simulink model "sixDOF_hw6"  (R2015a)
settings: Solver=ode113  StartTime=0.0  StopTime=t_total  MaxStep=60  MinStep=0.1  RelTol=1e-3
values from neighbouring files (symbols this model uses):
  A0 = zeros(3,3)    [PS2.m]    (also in PS3.m = getDCM(triad1, triad2); PS4.m = getDCM(triad1, triad2); PS5.m = getDCM(triad1, triad2); PS7.m = getDCM(triad1, triad2))
  a0 = 6776    [PS1.m]    (also in PS4.m; PS5.m; PS7.m)
  A_b2p = S_top.DCM_B2P    [PS5.m]    (also in PS7.m)
  b_perturbs = 1    [PS5.m]    (also in PS7.m; PS8.m; PS9.m)
  bGravGrad = 1    [PS1.m]    (also in PS4.m; PS5.m; PS7.m; PS8.m)
  bNoise = 1    [PS6.m]    (also in PS7.m; PS8.m = 0; PS9.m = 0)
  e0 = 0.0004758    [PS1.m]    (also in PS4.m; PS5.m; PS7.m)
  I_principle = S_top.tauCM_P    [PS2.m]    (also in PS3.m; PS4.m; PS5.m; PS7.m)
  incl0 = 51.6397    [PS1.m]    (also in PS4.m = 0; PS5.m = 0; PS7.m = 0)
  J2 = 0    [PS1.m]    (also in PS4.m; PS5.m; PS7.m)
  M0 = [0 0 0]'    [PS2.m]    (also in PS3.m; PS4.m; PS5.m; PS7.m)
  mu = 3.986e14 / 1000^3    (= 398600)    [PS1.m]    (also in PS4.m; PS5.m; PS7.m)
  normalsList = [normalsList, chd.normals]    [S_top2Lists.m]
  nu0 = 0    [PS1.m]    (also in PS4.m; PS5.m; PS7.m)
  OMEGA0 = 106.0758    [PS1.m]    (also in PS4.m = 0; PS5.m = 0; PS7.m = 0)
  omega0 = 233.6745    [PS1.m]    (also in PS4.m = 0; PS5.m = 0; PS7.m = 0)
  Re = 6371    [PS1.m]    (also in PS4.m; PS5.m; PS7.m)
  surfaceAreasList = [surfaceAreasList; chd.surfaceAreas]    [S_top2Lists.m]
  surfaceCM_bodyList = [surfaceCM_bodyList, chd.surfaceCM_body]    [S_top2Lists.m]
  tOffset = 0    [PS5.m]    (also in PS7.m)
  UTC_0 = [06,02,2017]    [PS5.m]    (also in PS7.m)
  w0 = w0_28    [PS2.m]    (also in PS3.m = [0; 0; 10/180*pi*rand()]; PS4.m = w0 + 0.0007*[1 1 1]'; PS5.m = [0 -n0 0]'; PS7.m = [0 -2 0]')
  wEarth = [0 0 7.292116e-5]'    [PS5.m]    (also in PS7.m)
settings Model: Creator=Toby  LastModifiedBy=Toby
settings DataIOCC: SaveTime=off

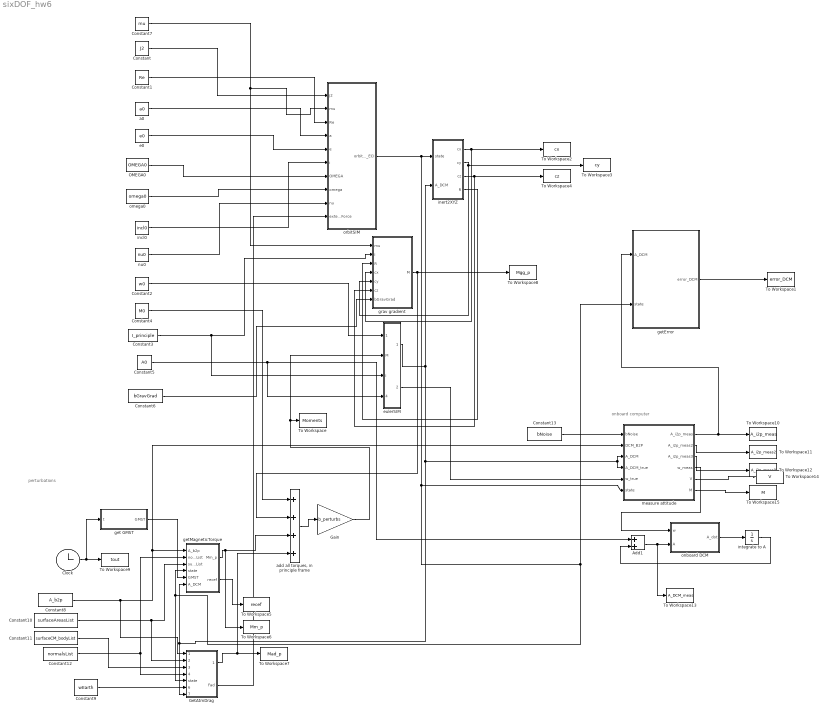
== system sixDOF_hw6 ==
  note: onboard computer
  note: perturbations
  Add1 : Sum
  Clock : Clock
  Constant : Constant  Value=J2
  Constant1 : Constant  Value=Re
  Constant10 : Constant  Value=surfaceAreasList
  Constant11 : Constant  Value=surfaceCM_bodyList
  Constant12 : Constant  Value=normalsList
  Constant13 : Constant  Value=bNoise
  Constant2 : Constant  Value=w0
  Constant3 : Constant  Value=I_principle
  Constant4 : Constant  Value=M0
  Constant5 : Constant  Value=A0
  Constant6 : Constant  Value=bGravGrad
  Constant7 : Constant  Value=mu
  Constant8 : Constant  Value=A_b2p
  Constant9 : Constant  Value=wEarth
  Gain : Gain  Gain=b_perturbs
  GetAtmDrag : MATLAB Function  TreatAsAtomicUnit=on
  OMEGA0 : Constant  Value=OMEGA0
  To Workspace : ToWorkspace  VariableName=Moments  SampleTime=-1
  To Workspace1 : ToWorkspace  VariableName=error_DCM  SampleTime=-1
  To Workspace10 : ToWorkspace  VariableName=A_i2p_meas  SampleTime=-1
  To Workspace11 : ToWorkspace  VariableName=A_i2p_meas2  SampleTime=-1
  To Workspace12 : ToWorkspace  VariableName=A_i2p_meas3  SampleTime=-1
  To Workspace13 : ToWorkspace  VariableName=A_DCM_meas  SampleTime=-1
  To Workspace14 : ToWorkspace  VariableName=V  SampleTime=-1
  To Workspace15 : ToWorkspace  VariableName=M  SampleTime=-1
  To Workspace2 : ToWorkspace  VariableName=cx  SampleTime=-1
  To Workspace3 : ToWorkspace  VariableName=cy  SampleTime=-1
  To Workspace4 : ToWorkspace  VariableName=cz  SampleTime=-1
  To Workspace5 : ToWorkspace  VariableName=recef  SampleTime=-1
  To Workspace6 : ToWorkspace  VariableName=Mm_p  SampleTime=-1
  To Workspace7 : ToWorkspace  VariableName=Mad_p  SampleTime=-1
  To Workspace8 : ToWorkspace  VariableName=Mgg_p  SampleTime=-1
  To Workspace9 : ToWorkspace  VariableName=tout  SampleTime=-1
  a0 : Constant  Value=a0
  "add all torques, in principle frame" : Sum  Inputs=++++
  e0 : Constant  Value=e0
  eulerSIM : Subsystem
  get GMST : Subsystem
  getError : MATLAB Function  TreatAsAtomicUnit=on
  getMagneticTorque : MATLAB Function  TreatAsAtomicUnit=on
  grav gradient : MATLAB Function  TreatAsAtomicUnit=on
  incl0 : Constant  Value=incl0
  inert2XYZ : MATLAB Function  TreatAsAtomicUnit=on
  integrate to A : Integrator
  measure attitude : MATLAB Function  TreatAsAtomicUnit=on
  nu0 : Constant  Value=nu0
  omega0 : Constant  Value=omega0
  onboard DCM : MATLAB Function  TreatAsAtomicUnit=on
  orbitSIM : Subsystem
  wires:
  Constant7/1 -> grav gradient/1(mu), orbitSIM/2(mu)
  Constant/1 -> orbitSIM/1(j2)
  Constant1/1 -> orbitSIM/3(Re)
  a0/1 -> orbitSIM/4(a)
  e0/1 -> orbitSIM/5(e)
  OMEGA0/1 -> orbitSIM/7(OMEGA)
  omega0/1 -> orbitSIM/8(omega)
  incl0/1 -> orbitSIM/6(i)
  nu0/1 -> orbitSIM/9(nu)
  Constant2/1 -> eulerSIM/1(w0)
  Constant3/1 -> grav gradient/2(I), eulerSIM/3(I)
  Constant5/1 -> Add1/1, eulerSIM/4(A0)
  inert2XYZ/1(cx) -> grav gradient/4(cx), To Workspace2/1
  inert2XYZ/2(cy) -> To Workspace3/1, grav gradient/5(cy)
  inert2XYZ/4(R) -> grav gradient/3(R)
  inert2XYZ/3(cz) -> To Workspace4/1, grav gradient/6(cz)
  Constant6/1 -> grav gradient/7(bGravGrad)
  Gain/1 -> eulerSIM/2(M), To Workspace/1
  GetAtmDrag/2(Fad) -> orbitSIM/10(externalForce)
  getError/1(error_DCM) -> To Workspace1/1
  grav gradient/1(M) -> "add all torques, in principle frame"/2, To Workspace8/1
  orbitSIM/1(orbit_state_ECI) -> measure attitude/6(state), getMagneticTorque/4(state), GetAtmDrag/5(state), getError/2(state), inert2XYZ/1(state)
  eulerSIM/1(A_DCM) -> inert2XYZ/2(A_DCM), measure attitude/4(A_DCM_true), measure attitude/3(A_DCM), getMagneticTorque/6(A_DCM), GetAtmDrag/7(A_DCM)
  "add all torques, in principle frame"/1 -> Gain/1
  Clock/1 -> get GMST/1(t), To Workspace9/1
  Constant8/1 -> measure attitude/2(DCM_B2P), getMagneticTorque/1(A_b2p), GetAtmDrag/1(A_b2p)
  GetAtmDrag/1(Mad_p) -> To Workspace7/1, "add all torques, in principle frame"/4
  Constant9/1 -> GetAtmDrag/6(wEarth)
  get GMST/1(GMST) -> getMagneticTorque/5(GMST)
  getMagneticTorque/2(recef) -> To Workspace5/1
  getMagneticTorque/1(Mm_p) -> "add all torques, in principle frame"/3, To Workspace6/1
  Constant12/1 -> getMagneticTorque/2(normalsList), GetAtmDrag/4(normalsList)
  Constant11/1 -> GetAtmDrag/3(surfaceCM_bodyList)
  Constant10/1 -> getMagneticTorque/3(surfaceAreasList), GetAtmDrag/2(surfaceAreasList)
  Constant4/1 -> "add all torques, in principle frame"/1
  onboard DCM/1(A_dot) -> integrate to A/1
  integrate to A/1 -> Add1/2
  Add1/1 -> To Workspace13/1, onboard DCM/2(A)
  measure attitude/4(w_meas) -> onboard DCM/1(w)
  measure attitude/1(A_i2p_meas) -> getError/1(A_DCM), To Workspace10/1
  measure attitude/2(A_i2p_meas2) -> To Workspace11/1
  measure attitude/3(A_i2p_meas3) -> To Workspace12/1
  Constant13/1 -> measure attitude/1(bNoise)
  eulerSIM/2(w_true) -> measure attitude/5(w_true)
  measure attitude/6(M) -> To Workspace15/1
  measure attitude/5(V) -> To Workspace14/1

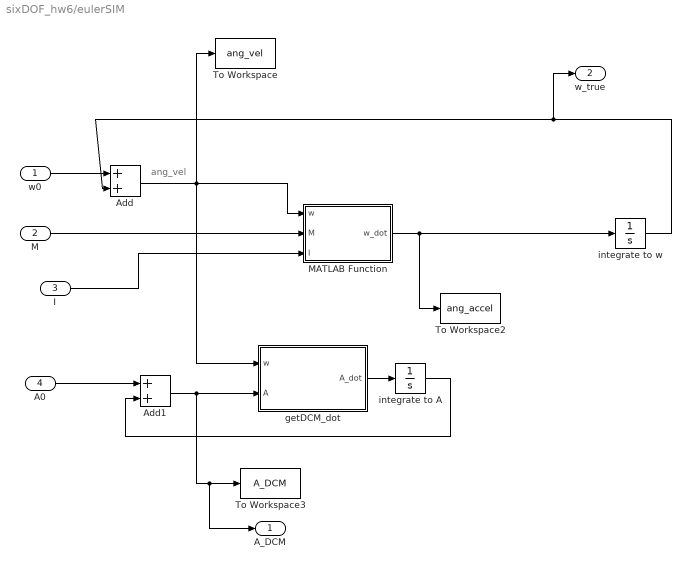
== system sixDOF_hw6/eulerSIM ==
  note: ang_vel
  w0 : Inport
  M : Inport  Port=2
  I : Inport  Port=3
  A0 : Inport  Port=4
  Add : Sum
  Add1 : Sum
  MATLAB Function : MATLAB Function  TreatAsAtomicUnit=on
  To Workspace : ToWorkspace  VariableName=ang_vel  SampleTime=-1
  To Workspace2 : ToWorkspace  VariableName=ang_accel  SampleTime=-1
  To Workspace3 : ToWorkspace  VariableName=A_DCM  SampleTime=-1
  getDCM_dot : MATLAB Function  TreatAsAtomicUnit=on
  integrate to A : Integrator
  integrate to w : Integrator
  A_DCM : Outport
  w_true : Outport  Port=2
  wires:
  w0/1 -> Add/1
  M/1 -> MATLAB Function/2(M)
  Add1/1 -> A_DCM/1, To Workspace3/1, getDCM_dot/2(A)
  I/1 -> MATLAB Function/3(I)
  getDCM_dot/1(A_dot) -> integrate to A/1
  A0/1 -> Add1/1
  integrate to A/1 -> Add1/2
  MATLAB Function/1(w_dot) -> integrate to w/1, To Workspace2/1
  integrate to w/1 -> w_true/1, Add/2
  Add/1 -> getDCM_dot/1(w), To Workspace/1, MATLAB Function/1(w)

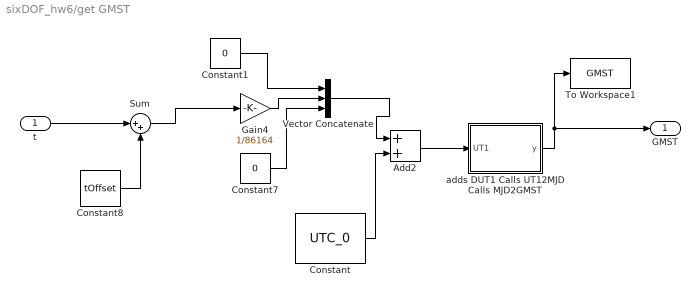
== system sixDOF_hw6/get GMST ==
  t : Inport
  Add2 : Sum
  Constant : Constant  Value=UTC_0
  Constant1 : Constant  Value=0
  Constant7 : Constant  Value=0
  Constant8 : Constant  Value=tOffset
  Gain4 : Gain  Gain=1/86164
  Sum : Sum  Inputs=|++
  To Workspace1 : ToWorkspace  VariableName=GMST  SampleTime=-1
  Vector Concatenate : Concatenate  NumInputs=3
  adds DUT1 Calls UT12MJD Calls MJD2GMST : MATLAB Function  TreatAsAtomicUnit=on
  GMST : Outport
  wires:
  Constant/1 -> Add2/2
  Constant7/1 -> Vector Concatenate/3
  Gain4/1 -> Vector Concatenate/2
  Constant1/1 -> Vector Concatenate/1
  Vector Concatenate/1 -> Add2/1
  Add2/1 -> adds DUT1 Calls UT12MJD Calls MJD2GMST/1(UT1)
  Sum/1 -> Gain4/1
  t/1 -> Sum/1
  Constant8/1 -> Sum/2
  adds DUT1 Calls UT12MJD Calls MJD2GMST/1(y) -> GMST/1, To Workspace1/1

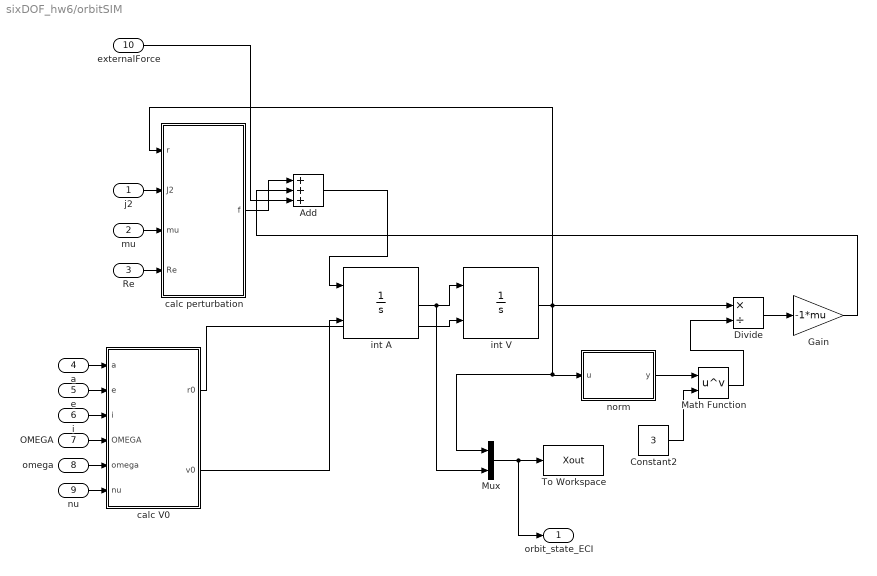
== system sixDOF_hw6/orbitSIM ==
  j2 : Inport
  mu : Inport  Port=2
  Re : Inport  Port=3
  a : Inport  Port=4
  e : Inport  Port=5
  i : Inport  Port=6
  OMEGA : Inport  Port=7
  omega : Inport  Port=8
  nu : Inport  Port=9
  externalForce : Inport  Port=10
  Add : Sum  Inputs=+++
  Constant2 : Constant  Value=3
  Divide : Product  Inputs=*/
  Gain : Gain  Gain=-1*mu
  Math Function : Math  Operator=pow  SaturateOnIntegerOverflow=on
  Mux : Mux  Inputs=2
  To Workspace : ToWorkspace  VariableName=Xout  SampleTime=-1
  calc V0 : MATLAB Function  TreatAsAtomicUnit=on
  calc perturbation : MATLAB Function  TreatAsAtomicUnit=on
  int A : Integrator  InitialConditionSource=external
  int V : Integrator  InitialConditionSource=external
  norm : MATLAB Function  TreatAsAtomicUnit=on
  orbit_state_ECI : Outport
  wires:
  calc V0/1(r0) -> int V/2
  Add/1 -> int A/1
  Mux/1 -> orbit_state_ECI/1, To Workspace/1
  norm/1(y) -> Math Function/1
  int V/1 -> calc perturbation/1(r), norm/1(u), Mux/1, Divide/1
  Math Function/1 -> Divide/2
  Divide/1 -> Gain/1
  Gain/1 -> Add/2
  calc V0/2(v0) -> int A/2
  int A/1 -> Mux/2, int V/1
  calc perturbation/1(f) -> Add/1
  Constant2/1 -> Math Function/2
  e/1 -> calc V0/2(e)
  i/1 -> calc V0/3(i)
  OMEGA/1 -> calc V0/4(OMEGA)
  a/1 -> calc V0/1(a)
  Re/1 -> calc perturbation/4(Re)
  mu/1 -> calc perturbation/3(mu)
  omega/1 -> calc V0/5(omega)
  j2/1 -> calc perturbation/2(J2)
  nu/1 -> calc V0/6(nu)
  externalForce/1 -> Add/3

== matlab function sixDOF_hw6/orbitSIM/norm ==
  data: u input; y output
function y = fcn(u)
%#codegen

y = norm(u);

== matlab function sixDOF_hw6/orbitSIM/calc perturbation ==
  data: r input; f output; J2 input; mu input; Re input
function f = fcn(r, J2, mu, Re)
% NOTE! EVERYTHING IN DEGREES
% 
% fR = -3*mu*J2*Re^2/(2*r^4)*(1-3*sind(incl)^2*sind(u)^2);
% fT = -3*mu*J2*Re^2/(2*r^4)*(sind(incl)^2*sind(u)*cosd(u));
% fN = -3*mu*J2*Re^2/(2*r^4)*(sind(incl)*cosd(incl)*sind(u));
rMag = norm(r);
rDir = r ./ norm(r);
f = -mu*J2*Re^2/2*( [0, 0, 6*r(3)/rMag^5]' + ...
      (3/rMag^4 - 15*(r(3)^2/rMag^6)).*rDir);

end

== matlab function sixDOF_hw6/orbitSIM/calc V0 ==
  data: a input; r0 output; e input; i input; OMEGA input; omega input; nu input; v0 output
function [r0, v0] = fcn(a, e, i, OMEGA, omega, nu)
%#codegen
[r0, v0] = OE2XV(a, e, i, OMEGA, omega, nu);
end

== matlab function sixDOF_hw6/getMagneticTorque ==
  data: A_b2p input; Mm_p output; normalsList input; surfaceAreasList input; state input; GMST input; A_DCM input; recef output
function [Mm_p, recef] = fcn(A_b2p, normalsList, surfaceAreasList, state, GMST, A_DCM)
%#codegen
xECI = state(1:3);
r = norm(xECI);
[ longitude, latitude, recef ] = getLongLatECEF( xECI, GMST );
coder.extrinsic('magneticTorque'); 
Mm_p = [0 0 0]';
[ Mm_p ] = magneticTorque( A_b2p, surfaceAreasList, normalsList, ...
  longitude, latitude, r, A_DCM, GMST);
end

== matlab function sixDOF_hw6/GetAtmDrag ==
  data: A_b2p input; Mad_p output; surfaceAreasList input; surfaceCM_bodyList input; normalsList input; state input; wEarth input; A_DCM input; Fad output
function [Mad_p, Fad] = fcn(A_b2p, surfaceAreasList, surfaceCM_bodyList, ...
  normalsList, state, wEarth, A_DCM)
%#codegen
xECI = state(1:3);
V_sc = state(4:6);
[ Fad, Mad ] = atmDragTorque(A_b2p, surfaceAreasList, surfaceCM_bodyList, ...
    normalsList, xECI, A_DCM, wEarth, V_sc );
A_p2i = getP2IfromA_DCM(A_DCM);
Mad_p = A_p2i' * Mad;
end

== matlab function sixDOF_hw6/getError ==
  data: A_DCM input; error_DCM output; state input
function error_DCM = fcn(A_DCM, state)
%#codegen
[ error_DCM ] = getAttError( A_DCM, state);

== matlab function sixDOF_hw6/eulerSIM/MATLAB Function ==
  data: w input; w_dot output; M input; I input
function w_dot = eulerRHS(w, M, I)
% principle axis euler eq
% w is 3x1 rotational velocity, expressed in principle
% M is 3x1 external torques, expressed in principle
Ix = I(1,1); Iy = I(2,2); Iz = I(3,3);
w_dot = zeros(3,1);
w_dot(1) = (M(1) - (Iz - Iy)*w(2)*w(3) ) / Ix;
w_dot(2) = (M(2) - (Ix - Iz)*w(1)*w(3) ) / Iy;
w_dot(3) = (M(3) - (Iy - Ix)*w(1)*w(2) ) / Iz;
end

== matlab function sixDOF_hw6/eulerSIM/getDCM_dot ==
  data: w input; A_dot output; A input
function A_dot   = getDCM_dot( w, A )
%GETDCM_DOT calculate time-derivative of DCM
% w is ang vel of body axes w.r.t. inertial EXPRESSED IN INERTIAL
[ A_dot ] = getDCM_dot( w, A );

end

== matlab function sixDOF_hw6/grav gradient ==
  data: mu input; M output; I input; R input; cx input; cy input; cz input; bGravGrad input
function M = fcn(mu, I, R, cx, cy, cz, bGravGrad)
%#codegen
if bGravGrad
  M = gravGradient( mu, I, R, cx, cy, cz );
else
  M = [0 0 0]';
end

== matlab function sixDOF_hw6/inert2XYZ ==
  data: cx output; state input; A_DCM input; cy output; cz output; R output
function [cx, cy, cz, R] = fcn(state, A_DCM)
%#codegen
%A should be principle to inertial
A = getP2IfromA_DCM( A_DCM );
R = norm(state(1:3));
c = 1 / R * A' * state(1:3);
cx = c(1);
cy = c(2);
cz = c(3);

== matlab function sixDOF_hw6/get GMST/adds DUT1 Calls UT12MJD Calls MJD2GMST ==
  data: UT1 input; y output
function y = fcn(UT1)
%u is calendar form
% DUT1= (UT1-UTC) transmitted with time signals                         
%              =  +0.5 seconds beginning 26 Jan 2017 at 0000 UTC  
UT1(2) = UT1(2) + 0.5; %defined offset
y1 = UT12MJD(UT1);
y = MJD2GMST(y1);

end

== matlab function sixDOF_hw6/measure attitude ==
  data: bNoise input; DCM_B2P input; A_i2p_meas output; A_DCM input; A_DCM_true input; w_true input; state input; A_i2p_meas2 output; A_i2p_meas3 output; w_meas output; V output; M output
function [ A_i2p_meas, A_i2p_meas2, A_i2p_meas3, w_meas, V,M ] = fcn( bNoise, DCM_B2P, A_DCM, A_DCM_true, w_true, state )
%#codegen
[ A_i2p_meas, A_i2p_meas2, A_i2p_meas3, V, M ] = measureAtt( bNoise, DCM_B2P, A_DCM, A_DCM_true, state );
w_meas = measureOMEGA(w_true, DCM_B2P, bNoise);

== matlab function sixDOF_hw6/onboard DCM ==
  data: w input; A_dot output; A input
function A_dot   = getDCM_dot( w, A )
%GETDCM_DOT calculate time-derivative of DCM
% w is ang vel of body axes w.r.t. inertial EXPRESSED IN INERTIAL
[ A_dot ] = getDCM_dot( w, A );

end
